simulink model "lab2_2"  (R2023b)
settings: Solver=VariableStepAuto  StartTime=0.0  StopTime=50.0  MaxStep=2^-7  RelTol=1e-3
settings Model: Creator=insomnia  LastModifiedBy=insomnia

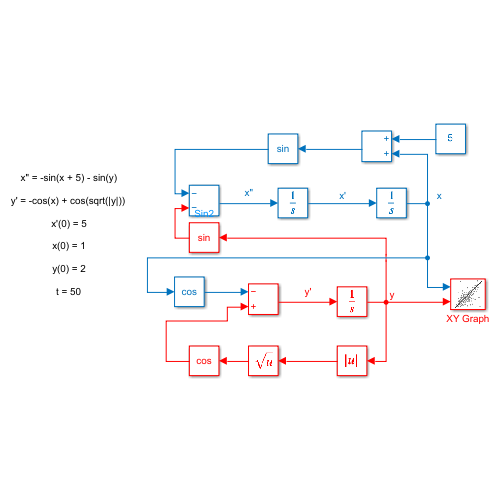
[thumbnail: Simulink's stored preview of the top-level diagram]
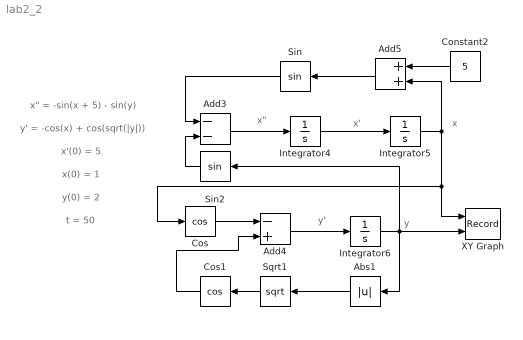
== system lab2_2 ==
  note: y'
  note: t = 50
  note: x
  note: x'(0) = 5
  note: x'
  note: y
  note: x" = -sin(x + 5) - sin(y)
  note: x(0) = 1
  note: x"
  note: y' = -cos(x) + cos(sqrt(|y|))
  note: y(0) = 2
  Abs1 : Abs  SaturateOnIntegerOverflow=off
  Add3 : Sum  Inputs=--
  Add4 : Sum  Inputs=-+
  Add5 : Sum
  Constant2 : Constant  Value=5
  Cos : Trigonometry  Operator=cos
  Cos1 : Trigonometry  Operator=cos
  Integrator4 : Integrator  InitialCondition=5
  Integrator5 : Integrator  InitialCondition=1
  Integrator6 : Integrator  InitialCondition=2
  Sin : Trigonometry
  Sin2 : Trigonometry
  Sqrt1 : Sqrt
  XY Graph : Record  FileSettingsInternal="{\"entries\":[{\"content\":{\"excelSettings\":{\"content\":{},\"type\":\"Streamout.ExcelSettings\"}},\"type\":\"Streamout.FileSettingStorage\",\"uuid\":\"\"}],\"packageUris\":[\"http:\\/\\/schema.mathworks.com\\/mf0\\/streamout_blocks\\/R2020a\"],\"version\":\"1.0\"}"  Layout=[1 1]  SignalsInternal="{\"entries\":[{\"content\":{\"signals\":[{\"content\":{\"blockPath\":[],\"dimensions\":[1],\"domain\":\"\",\"lineColor\":\"#a2142f\",\"plots\":[ 1 ],\"port\":1,\"signalID\":1,\"signalName\":\"Integrator5\"},\"type\":\"RecordBlkView.Signal\",\"uuid\":\"\"},{\"content\":{\"blockPath\":[],\"dimensions\":[1],\"domain\":\"\",\"lineColor\":\"#139fff\",\"plots\":[ 1 ],\"port\":2,\"signalID\":2,\"signalName\":\"Integrator6\"},\"type\":\"RecordBlkView.Signal\",\"uuid\":\"\"}]},\"type\":\"RecordBlkView.InputSignals\",\"uuid\":\"\"}],\"packageUris\":[\"http:\\/\\/schema.mathworks.com\\/mf0\\/streamout_blocks\\/R2020a\"],\"version\":\"1.0\"}"  VisualizationBindings="{\"xyplotplugin\":{\"info\":[{\"series\":[{\"bindingParametersList\":[{\"parameter\":\"X-Axis\",\"signalID\":1,\"signalName\":\"Integrator5\"},{\"parameter\":\"Y-Axis\",\"signalID\":2,\"signalName\":\"Integrator6\"}],\"seriesID\":0}],\"subplotID\":1}]}}"  CompatibilityTag=XY
  wires:
  Abs1/1 -> Sqrt1/1
  Constant2/1 -> Add5/1
  Add5/1 -> Sin/1
  Cos1/1 -> Add4/2
  Sqrt1/1 -> Cos1/1
  Integrator6/1 -> Sin2/1, XY Graph/2, Abs1/1
  Sin/1 -> Add3/1
  Add3/1 -> Integrator4/1
  Integrator4/1 -> Integrator5/1
  Cos/1 -> Add4/1
  Integrator5/1 -> Cos/1, XY Graph/1, Add5/2
  Sin2/1 -> Add3/2
  Add4/1 -> Integrator6/1
